simulink model "alternative_agent_model"  (R2020b)
settings: Solver=VariableStepAuto  StartTime=0.0  StopTime=10.0  RelTol=1e-3
values from neighbouring files (symbols this model uses):
  A = A_plant - B_plant*K_plant    [alternative_model.m]    (also in alternative_model_script.m; free_response.m = sym('A', [2,2]); p1.m; stable_template.m)
  A_plant = [0 1; 880.87 0]    [alternative_model.m]    (also in alternative_model_script.m; observer_convergence.m = A_plant - B_plant * K; p1.m; stable_template.m)
  B_plant = [0; -9.9453]    [alternative_model.m]    (also in alternative_model_script.m; observer_convergence.m; p1.m; stable_template.m)
  c = 10/den    [alternative_model.m]    (also in alternative_model_script.m; p1.m = 100/den; stable_template.m; template.m)
  C = C_plant    [alternative_model.m]    (also in alternative_model_script.m; free_response.m = sym('C', [1,2]); p1.m; stable_template.m)
  C_plant = [708.27 0]    [alternative_model.m]    (also in alternative_model_script.m; observer_convergence.m; p1.m; stable_template.m)
  F = P * C' / R    [alternative_model.m]    (also in alternative_model_script.m; observer_convergence.m = P * C_plant' / R; p1.m; stable_template.m)
  K = B'/R*P    [alternative_model.m]    (also in alternative_model_script.m; free_response.m = sym('K', [2,2]); observer_convergence.m = acker(A_plant, B_plant, [0 0]); p1.m)
  K_plant = acker(A_plant, B_plant, poles)    [alternative_model.m]    (also in alternative_model_script.m; p1.m; stable_template.m; template.m)
  output_state = 1    [v1.m]
  x0_agent = [0.1 2]    [alternative_model.m]    (also in alternative_model_script.m; p1.m = [0 0]; stable_template.m = [0 0]; template.m = [0 0])
libraries: simulink x1
settings Model: Creator=salvo  LastModifiedBy=salvo
settings ModelReferenceCC: ModelReferenceMinAlgLoopOccurrences=on

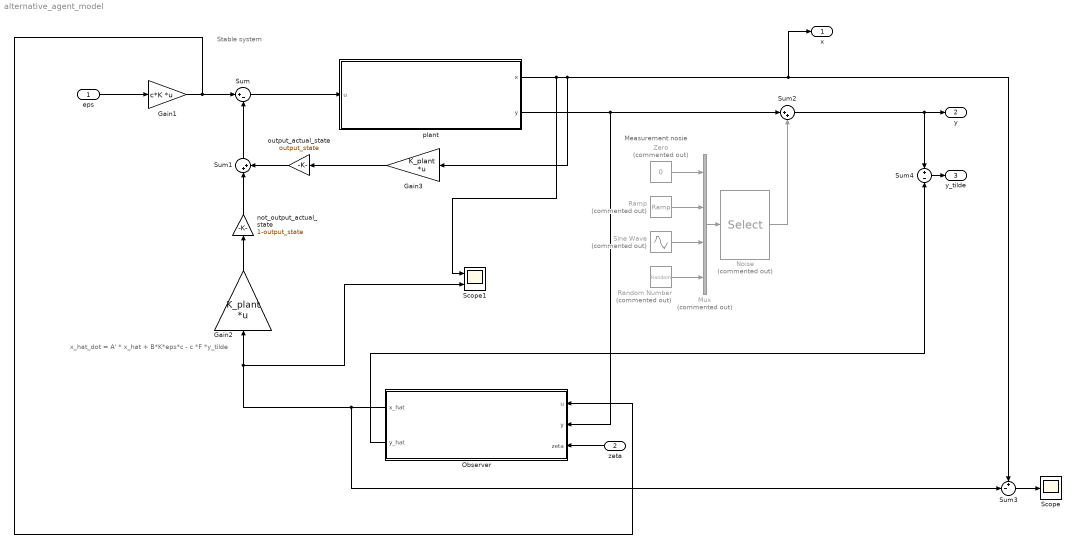
== system alternative_agent_model ==
  note: x_hat_dot = A' * x_hat + B*K*eps*c - c *F *y_tilde
  note: Stable system
  note: Measurement nosie
  eps : Inport  PortDimensions=[2, 1]
  zeta : Inport  Port=2
  Gain1 : Gain  Gain=c*K  Multiplication=Matrix(K*u)
  Gain2 : Gain  Gain=K_plant  Multiplication=Matrix(K*u)
  Gain3 : Gain  Gain=K_plant  Multiplication=Matrix(K*u)
  Mux : Mux  Commented=on
  Noise : Selector  Commented=on  InputPortWidth=4  IndexOptions=Index vector (dialog)  Indices=measurement_noise_type  OutputSizes=1
  Observer : Subsystem
  Ramp : simulink/Sources/Ramp  Commented=on  slope=1  start=0  InitialOutput=0
  Random Number : RandomNumber  Commented=on  SampleTime=0.1
  Scope : Scope
  Scope1 : Scope  NumInputPorts=2
  Sine Wave : Sin  Commented=on  SampleTime=0
  Sum : Sum  Inputs=|+-
  Sum1 : Sum  Inputs=|++
  Sum2 : Sum  Inputs=|++
  Sum3 : Sum  Inputs=+-|
  Sum4 : Sum  Inputs=+-
  Zero : Constant  Commented=on  Value=0  OutDataTypeStr=Inherit: Inherit via back propagation
  not_output_actual_state : Gain  Gain=1-output_state
  output_actual_state : Gain  Gain=output_state
  plant : Subsystem
  x : Outport
  y : Outport  Port=2
  y_tilde : Outport  Port=3  PortDimensions=1
  wires:
  zeta/1 -> Observer/3(zeta)
  eps/1 -> Gain1/1
  plant/1(x) -> Scope1/1, Gain3/1, x/1, Sum3/1
  Gain1/1 -> Sum/1, Observer/1(u)
  Gain3/1 -> output_actual_state/1
  plant/2(y) -> Observer/2(y), Sum2/1
  Zero/1 -> Mux/1
  Noise/1 -> Sum2/2
  Sum2/1 -> Sum4/1, y/1
  Random Number/1 -> Mux/4
  Ramp/1 -> Mux/2
  Sine Wave/1 -> Mux/3
  Mux/1 -> Noise/1
  Sum3/1 -> Scope/1
  Observer/2(y_hat) -> Sum4/2
  Sum4/1 -> y_tilde/1
  Sum/1 -> plant/1(u)
  Observer/1(x_hat) -> Sum3/2, Gain2/1, Scope1/2
  Gain2/1 -> not_output_actual_state/1
  not_output_actual_state/1 -> Sum1/1
  output_actual_state/1 -> Sum1/2
  Sum1/1 -> Sum/2

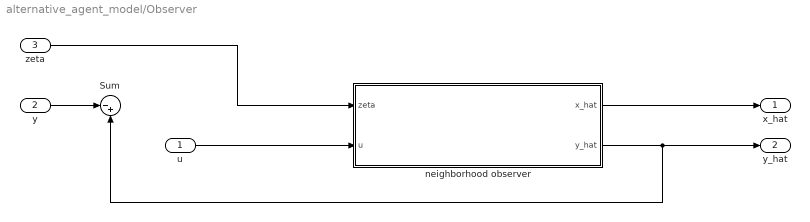
== system alternative_agent_model/Observer ==
  u : Inport
  y : Inport  Port=2
  zeta : Inport  Port=3
  Sum : Sum  Inputs=|-+
  neighborhood observer : Subsystem
  x_hat : Outport  PortDimensions=[2 1]
  y_hat : Outport  Port=2
  wires:
  u/1 -> neighborhood observer/2(u)
  neighborhood observer/1(x_hat) -> x_hat/1
  neighborhood observer/2(y_hat) -> Sum/2, y_hat/1
  y/1 -> Sum/1
  zeta/1 -> neighborhood observer/1(zeta)

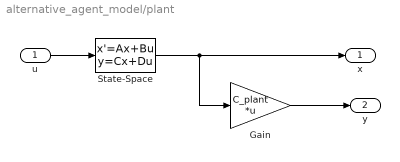
== system alternative_agent_model/plant ==
  u : Inport
  Gain : Gain  Gain=C_plant  Multiplication=Matrix(K*u)
  State-Space : StateSpace  A=A_plant  B=B_plant  C=eye(2)  D=[0; 0]  InitialCondition=x0_agent
  x : Outport
  y : Outport  Port=2  PortDimensions=1
  wires:
  u/1 -> State-Space/1
  Gain/1 -> y/1
  State-Space/1 -> x/1, Gain/1

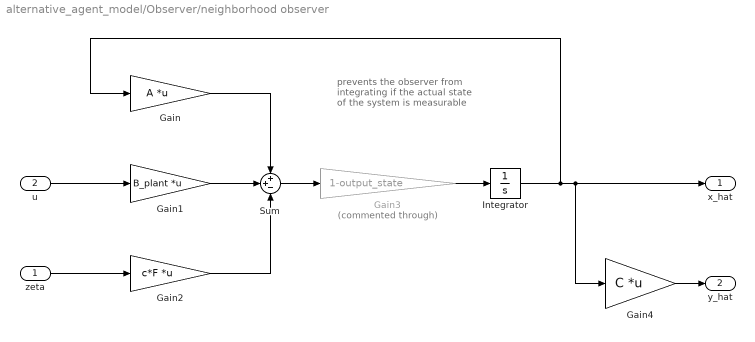
== system alternative_agent_model/Observer/neighborhood observer ==
  note: prevents the observer from integrating if the actual state of the system is measurable
  zeta : Inport
  u : Inport  Port=2
  Gain : Gain  Gain=A  Multiplication=Matrix(K*u)
  Gain1 : Gain  Gain=B_plant  Multiplication=Matrix(K*u)
  Gain2 : Gain  Gain=c*F  Multiplication=Matrix(K*u)
  Gain3 : Gain  Commented=through  Gain=1-output_state
  Gain4 : Gain  Gain=C  Multiplication=Matrix(K*u)
  Integrator : Integrator
  Sum : Sum  Inputs=++-
  x_hat : Outport
  y_hat : Outport  Port=2
  wires:
  Integrator/1 -> Gain/1, x_hat/1, Gain4/1
  Gain/1 -> Sum/1
  Gain1/1 -> Sum/2
  u/1 -> Gain1/1
  Gain2/1 -> Sum/3
  zeta/1 -> Gain2/1
  Sum/1 -> Gain3/1
  Gain3/1 -> Integrator/1
  Gain4/1 -> y_hat/1
